simulink model "fourteen_bus_linear_network"  (R2020b)
settings: Solver=VariableStepAuto  StartTime=0.0  StopTime=1.000000  RelTol=1e-3
libraries: powerlib x124, powerlib_meascontrol x2
(part 2 of 2)

== system fourteen_bus_linear_network/Subsystem6 ==
  From Workspace15 : FromWorkspace  VariableName=load14_Ia_ts
  From Workspace16 : FromWorkspace  VariableName=load14_Ib_ts
  From Workspace17 : FromWorkspace  VariableName=load14_Ic_ts
  Subsystem3 : Subsystem
  A : PMIOPort  Side=Right
  B : PMIOPort  Port=2  Side=Right
  C : PMIOPort  Port=3  Side=Right
  wires:
  From Workspace15/1 -> Subsystem3/1(Ia)
  From Workspace17/1 -> Subsystem3/3(Ic)
  From Workspace16/1 -> Subsystem3/2(Ib)
  connections:
  Subsystem3/RConn2 -- B/RConn1
  Subsystem3/RConn1 -- A/RConn1
  Subsystem3/RConn3 -- C/RConn1

== system fourteen_bus_linear_network/Subsystem7 ==
  From Workspace15 : FromWorkspace  VariableName=load6_Ia_ts
  From Workspace16 : FromWorkspace  VariableName=load6_Ib_ts
  From Workspace17 : FromWorkspace  VariableName=load6_Ic_ts
  Subsystem3 : Subsystem
  A : PMIOPort  Side=Right
  B : PMIOPort  Port=2  Side=Right
  C : PMIOPort  Port=3  Side=Right
  wires:
  From Workspace15/1 -> Subsystem3/1(Ia)
  From Workspace17/1 -> Subsystem3/3(Ic)
  From Workspace16/1 -> Subsystem3/2(Ib)
  connections:
  Subsystem3/RConn2 -- B/RConn1
  Subsystem3/RConn1 -- A/RConn1
  Subsystem3/RConn3 -- C/RConn1

== system fourteen_bus_linear_network/Subsystem8 ==
  From Workspace15 : FromWorkspace  VariableName=load13_Ia_ts
  From Workspace16 : FromWorkspace  VariableName=load13_Ib_ts
  From Workspace17 : FromWorkspace  VariableName=load13_Ic_ts
  Subsystem3 : Subsystem
  A : PMIOPort  Side=Right
  B : PMIOPort  Port=2  Side=Right
  C : PMIOPort  Port=3  Side=Right
  wires:
  From Workspace15/1 -> Subsystem3/1(Ia)
  From Workspace17/1 -> Subsystem3/3(Ic)
  From Workspace16/1 -> Subsystem3/2(Ib)
  connections:
  Subsystem3/RConn2 -- B/RConn1
  Subsystem3/RConn1 -- A/RConn1
  Subsystem3/RConn3 -- C/RConn1

== system fourteen_bus_linear_network/Subsystem9 ==
  From Workspace15 : FromWorkspace  VariableName=load12_Ia_ts
  From Workspace16 : FromWorkspace  VariableName=load12_Ib_ts
  From Workspace17 : FromWorkspace  VariableName=load12_Ic_ts
  Subsystem3 : Subsystem
  A : PMIOPort  Side=Right
  B : PMIOPort  Port=2  Side=Right
  C : PMIOPort  Port=3  Side=Right
  wires:
  From Workspace15/1 -> Subsystem3/1(Ia)
  From Workspace17/1 -> Subsystem3/3(Ic)
  From Workspace16/1 -> Subsystem3/2(Ib)
  connections:
  Subsystem3/RConn2 -- B/RConn1
  Subsystem3/RConn1 -- A/RConn1
  Subsystem3/RConn3 -- C/RConn1

== system fourteen_bus_linear_network/Subsystem1/Subsystem1 ==
  Ia : Inport
  Ib : Inport  Port=2
  Ic : Inport  Port=3
  Controlled Current Source10 : powerlib/Electrical Sources/Controlled Current Source  Initialize=on  Source_Type=AC  Amplitude=0  Phase=0  Frequency=0  Measurements=None
  Controlled Current Source11 : powerlib/Electrical Sources/Controlled Current Source  Initialize=on  Source_Type=AC  Amplitude=0  Phase=0  Frequency=0  Measurements=None
  Controlled Current Source9 : powerlib/Electrical Sources/Controlled Current Source  Initialize=on  Source_Type=AC  Amplitude=0  Phase=0  Frequency=0  Measurements=None
  Ground2 : powerlib/Elements/Ground  LConnTagsString=a
  A : PMIOPort  Side=Right
  B : PMIOPort  Port=2  Side=Right
  C : PMIOPort  Port=3  Side=Right
  wires:
  Ia/1 -> Controlled Current Source9/1
  Ic/1 -> Controlled Current Source11/1
  Ib/1 -> Controlled Current Source10/1
  connections:
  Controlled Current Source10/RConn1 -- B/RConn1
  Controlled Current Source9/RConn1 -- A/RConn1
  Controlled Current Source11/RConn1 -- C/RConn1
  Controlled Current Source11/LConn1 -- Controlled Current Source10/LConn1 -- Controlled Current Source9/LConn1 -- Ground2/LConn1

== system fourteen_bus_linear_network/Subsystem10/Subsystem3 ==
  Ia : Inport
  Ib : Inport  Port=2
  Ic : Inport  Port=3
  Controlled Current Source10 : powerlib/Electrical Sources/Controlled Current Source  Initialize=on  Source_Type=AC  Amplitude=0  Phase=0  Frequency=0  Measurements=None
  Controlled Current Source11 : powerlib/Electrical Sources/Controlled Current Source  Initialize=on  Source_Type=AC  Amplitude=0  Phase=0  Frequency=0  Measurements=None
  Controlled Current Source9 : powerlib/Electrical Sources/Controlled Current Source  Initialize=on  Source_Type=AC  Amplitude=0  Phase=0  Frequency=0  Measurements=None
  Ground2 : powerlib/Elements/Ground  LConnTagsString=a
  A : PMIOPort  Side=Right
  B : PMIOPort  Port=2  Side=Right
  C : PMIOPort  Port=3  Side=Right
  wires:
  Ia/1 -> Controlled Current Source9/1
  Ic/1 -> Controlled Current Source11/1
  Ib/1 -> Controlled Current Source10/1
  connections:
  Controlled Current Source10/RConn1 -- B/RConn1
  Controlled Current Source9/RConn1 -- A/RConn1
  Controlled Current Source11/RConn1 -- C/RConn1
  Controlled Current Source10/LConn1 -- Controlled Current Source11/LConn1 -- Controlled Current Source9/LConn1 -- Ground2/LConn1

== system fourteen_bus_linear_network/Subsystem11/Subsystem3 ==
  Ia : Inport
  Ib : Inport  Port=2
  Ic : Inport  Port=3
  Controlled Current Source10 : powerlib/Electrical Sources/Controlled Current Source  Initialize=on  Source_Type=AC  Amplitude=0  Phase=0  Frequency=0  Measurements=None
  Controlled Current Source11 : powerlib/Electrical Sources/Controlled Current Source  Initialize=on  Source_Type=AC  Amplitude=0  Phase=0  Frequency=0  Measurements=None
  Controlled Current Source9 : powerlib/Electrical Sources/Controlled Current Source  Initialize=on  Source_Type=AC  Amplitude=0  Phase=0  Frequency=0  Measurements=None
  Ground2 : powerlib/Elements/Ground  LConnTagsString=a
  A : PMIOPort  Side=Right
  B : PMIOPort  Port=2  Side=Right
  C : PMIOPort  Port=3  Side=Right
  wires:
  Ia/1 -> Controlled Current Source9/1
  Ic/1 -> Controlled Current Source11/1
  Ib/1 -> Controlled Current Source10/1
  connections:
  Controlled Current Source10/RConn1 -- B/RConn1
  Controlled Current Source9/RConn1 -- A/RConn1
  Controlled Current Source11/RConn1 -- C/RConn1
  Controlled Current Source10/LConn1 -- Controlled Current Source11/LConn1 -- Controlled Current Source9/LConn1 -- Ground2/LConn1

== system fourteen_bus_linear_network/Subsystem12/Subsystem1 ==
  Ia : Inport
  Ib : Inport  Port=2
  Ic : Inport  Port=3
  Controlled Current Source10 : powerlib/Electrical Sources/Controlled Current Source  Initialize=on  Source_Type=AC  Amplitude=0  Phase=0  Frequency=0  Measurements=None
  Controlled Current Source11 : powerlib/Electrical Sources/Controlled Current Source  Initialize=on  Source_Type=AC  Amplitude=0  Phase=0  Frequency=0  Measurements=None
  Controlled Current Source9 : powerlib/Electrical Sources/Controlled Current Source  Initialize=on  Source_Type=AC  Amplitude=0  Phase=0  Frequency=0  Measurements=None
  Ground2 : powerlib/Elements/Ground  LConnTagsString=a
  A : PMIOPort  Side=Right
  B : PMIOPort  Port=2  Side=Right
  C : PMIOPort  Port=3  Side=Right
  wires:
  Ia/1 -> Controlled Current Source9/1
  Ic/1 -> Controlled Current Source11/1
  Ib/1 -> Controlled Current Source10/1
  connections:
  Controlled Current Source10/RConn1 -- B/RConn1
  Controlled Current Source9/RConn1 -- A/RConn1
  Controlled Current Source11/RConn1 -- C/RConn1
  Controlled Current Source11/LConn1 -- Ground2/LConn1 -- Controlled Current Source10/LConn1 -- Controlled Current Source9/LConn1

== system fourteen_bus_linear_network/Subsystem13/Subsystem1 ==
  Ia : Inport
  Ib : Inport  Port=2
  Ic : Inport  Port=3
  Controlled Current Source10 : powerlib/Electrical Sources/Controlled Current Source  Initialize=on  Source_Type=AC  Amplitude=0  Phase=0  Frequency=0  Measurements=None
  Controlled Current Source11 : powerlib/Electrical Sources/Controlled Current Source  Initialize=on  Source_Type=AC  Amplitude=0  Phase=0  Frequency=0  Measurements=None
  Controlled Current Source9 : powerlib/Electrical Sources/Controlled Current Source  Initialize=on  Source_Type=AC  Amplitude=0  Phase=0  Frequency=0  Measurements=None
  Ground2 : powerlib/Elements/Ground  LConnTagsString=a
  A : PMIOPort  Side=Right
  B : PMIOPort  Port=2  Side=Right
  C : PMIOPort  Port=3  Side=Right
  wires:
  Ia/1 -> Controlled Current Source9/1
  Ic/1 -> Controlled Current Source11/1
  Ib/1 -> Controlled Current Source10/1
  connections:
  Controlled Current Source10/RConn1 -- B/RConn1
  Controlled Current Source9/RConn1 -- A/RConn1
  Controlled Current Source11/RConn1 -- C/RConn1
  Controlled Current Source11/LConn1 -- Controlled Current Source10/LConn1 -- Controlled Current Source9/LConn1 -- Ground2/LConn1

== system fourteen_bus_linear_network/Subsystem3/Subsystem3 ==
  Ia : Inport
  Ib : Inport  Port=2
  Ic : Inport  Port=3
  Controlled Current Source10 : powerlib/Electrical Sources/Controlled Current Source  Initialize=on  Source_Type=AC  Amplitude=0  Phase=0  Frequency=0  Measurements=None
  Controlled Current Source11 : powerlib/Electrical Sources/Controlled Current Source  Initialize=on  Source_Type=AC  Amplitude=0  Phase=0  Frequency=0  Measurements=None
  Controlled Current Source9 : powerlib/Electrical Sources/Controlled Current Source  Initialize=on  Source_Type=AC  Amplitude=0  Phase=0  Frequency=0  Measurements=None
  Ground2 : powerlib/Elements/Ground  LConnTagsString=a
  A : PMIOPort  Side=Right
  B : PMIOPort  Port=2  Side=Right
  C : PMIOPort  Port=3  Side=Right
  wires:
  Ia/1 -> Controlled Current Source9/1
  Ic/1 -> Controlled Current Source11/1
  Ib/1 -> Controlled Current Source10/1
  connections:
  Controlled Current Source10/RConn1 -- B/RConn1
  Controlled Current Source9/RConn1 -- A/RConn1
  Controlled Current Source11/RConn1 -- C/RConn1
  Controlled Current Source10/LConn1 -- Controlled Current Source11/LConn1 -- Controlled Current Source9/LConn1 -- Ground2/LConn1

== system fourteen_bus_linear_network/Subsystem4/Subsystem3 ==
  Ia : Inport
  Ib : Inport  Port=2
  Ic : Inport  Port=3
  Controlled Current Source10 : powerlib/Electrical Sources/Controlled Current Source  Initialize=on  Source_Type=AC  Amplitude=0  Phase=0  Frequency=0  Measurements=None
  Controlled Current Source11 : powerlib/Electrical Sources/Controlled Current Source  Initialize=on  Source_Type=AC  Amplitude=0  Phase=0  Frequency=0  Measurements=None
  Controlled Current Source9 : powerlib/Electrical Sources/Controlled Current Source  Initialize=on  Source_Type=AC  Amplitude=0  Phase=0  Frequency=0  Measurements=None
  Ground2 : powerlib/Elements/Ground  LConnTagsString=a
  A : PMIOPort  Side=Right
  B : PMIOPort  Port=2  Side=Right
  C : PMIOPort  Port=3  Side=Right
  wires:
  Ia/1 -> Controlled Current Source9/1
  Ic/1 -> Controlled Current Source11/1
  Ib/1 -> Controlled Current Source10/1
  connections:
  Controlled Current Source10/RConn1 -- B/RConn1
  Controlled Current Source9/RConn1 -- A/RConn1
  Controlled Current Source11/RConn1 -- C/RConn1
  Controlled Current Source10/LConn1 -- Controlled Current Source11/LConn1 -- Controlled Current Source9/LConn1 -- Ground2/LConn1

== system fourteen_bus_linear_network/Subsystem5/Subsystem3 ==
  Ia : Inport
  Ib : Inport  Port=2
  Ic : Inport  Port=3
  Controlled Current Source10 : powerlib/Electrical Sources/Controlled Current Source  Initialize=on  Source_Type=AC  Amplitude=0  Phase=0  Frequency=0  Measurements=None
  Controlled Current Source11 : powerlib/Electrical Sources/Controlled Current Source  Initialize=on  Source_Type=AC  Amplitude=0  Phase=0  Frequency=0  Measurements=None
  Controlled Current Source9 : powerlib/Electrical Sources/Controlled Current Source  Initialize=on  Source_Type=AC  Amplitude=0  Phase=0  Frequency=0  Measurements=None
  Ground2 : powerlib/Elements/Ground  LConnTagsString=a
  A : PMIOPort  Side=Right
  B : PMIOPort  Port=2  Side=Right
  C : PMIOPort  Port=3  Side=Right
  wires:
  Ia/1 -> Controlled Current Source9/1
  Ic/1 -> Controlled Current Source11/1
  Ib/1 -> Controlled Current Source10/1
  connections:
  Controlled Current Source10/RConn1 -- B/RConn1
  Controlled Current Source9/RConn1 -- A/RConn1
  Controlled Current Source11/RConn1 -- C/RConn1
  Controlled Current Source11/LConn1 -- Controlled Current Source10/LConn1 -- Ground2/LConn1 -- Controlled Current Source9/LConn1

== system fourteen_bus_linear_network/Subsystem6/Subsystem3 ==
  Ia : Inport
  Ib : Inport  Port=2
  Ic : Inport  Port=3
  Controlled Current Source10 : powerlib/Electrical Sources/Controlled Current Source  Initialize=on  Source_Type=AC  Amplitude=0  Phase=0  Frequency=0  Measurements=None
  Controlled Current Source11 : powerlib/Electrical Sources/Controlled Current Source  Initialize=on  Source_Type=AC  Amplitude=0  Phase=0  Frequency=0  Measurements=None
  Controlled Current Source9 : powerlib/Electrical Sources/Controlled Current Source  Initialize=on  Source_Type=AC  Amplitude=0  Phase=0  Frequency=0  Measurements=None
  Ground2 : powerlib/Elements/Ground  LConnTagsString=a
  A : PMIOPort  Side=Right
  B : PMIOPort  Port=2  Side=Right
  C : PMIOPort  Port=3  Side=Right
  wires:
  Ia/1 -> Controlled Current Source9/1
  Ic/1 -> Controlled Current Source11/1
  Ib/1 -> Controlled Current Source10/1
  connections:
  Controlled Current Source10/RConn1 -- B/RConn1
  Controlled Current Source9/RConn1 -- A/RConn1
  Controlled Current Source11/RConn1 -- C/RConn1
  Controlled Current Source10/LConn1 -- Controlled Current Source11/LConn1 -- Controlled Current Source9/LConn1 -- Ground2/LConn1

== system fourteen_bus_linear_network/Subsystem7/Subsystem3 ==
  Ia : Inport
  Ib : Inport  Port=2
  Ic : Inport  Port=3
  Controlled Current Source10 : powerlib/Electrical Sources/Controlled Current Source  Initialize=on  Source_Type=AC  Amplitude=0  Phase=0  Frequency=0  Measurements=None
  Controlled Current Source11 : powerlib/Electrical Sources/Controlled Current Source  Initialize=on  Source_Type=AC  Amplitude=0  Phase=0  Frequency=0  Measurements=None
  Controlled Current Source9 : powerlib/Electrical Sources/Controlled Current Source  Initialize=on  Source_Type=AC  Amplitude=0  Phase=0  Frequency=0  Measurements=None
  Ground2 : powerlib/Elements/Ground  LConnTagsString=a
  A : PMIOPort  Side=Right
  B : PMIOPort  Port=2  Side=Right
  C : PMIOPort  Port=3  Side=Right
  wires:
  Ia/1 -> Controlled Current Source9/1
  Ic/1 -> Controlled Current Source11/1
  Ib/1 -> Controlled Current Source10/1
  connections:
  Controlled Current Source10/RConn1 -- B/RConn1
  Controlled Current Source9/RConn1 -- A/RConn1
  Controlled Current Source11/RConn1 -- C/RConn1
  Controlled Current Source10/LConn1 -- Controlled Current Source11/LConn1 -- Controlled Current Source9/LConn1 -- Ground2/LConn1

== system fourteen_bus_linear_network/Subsystem8/Subsystem3 ==
  Ia : Inport
  Ib : Inport  Port=2
  Ic : Inport  Port=3
  Controlled Current Source10 : powerlib/Electrical Sources/Controlled Current Source  Initialize=on  Source_Type=AC  Amplitude=0  Phase=0  Frequency=0  Measurements=None
  Controlled Current Source11 : powerlib/Electrical Sources/Controlled Current Source  Initialize=on  Source_Type=AC  Amplitude=0  Phase=0  Frequency=0  Measurements=None
  Controlled Current Source9 : powerlib/Electrical Sources/Controlled Current Source  Initialize=on  Source_Type=AC  Amplitude=0  Phase=0  Frequency=0  Measurements=None
  Ground2 : powerlib/Elements/Ground  LConnTagsString=a
  A : PMIOPort  Side=Right
  B : PMIOPort  Port=2  Side=Right
  C : PMIOPort  Port=3  Side=Right
  wires:
  Ia/1 -> Controlled Current Source9/1
  Ic/1 -> Controlled Current Source11/1
  Ib/1 -> Controlled Current Source10/1
  connections:
  Controlled Current Source10/RConn1 -- B/RConn1
  Controlled Current Source9/RConn1 -- A/RConn1
  Controlled Current Source11/RConn1 -- C/RConn1
  Controlled Current Source10/LConn1 -- Controlled Current Source11/LConn1 -- Controlled Current Source9/LConn1 -- Ground2/LConn1

== system fourteen_bus_linear_network/Subsystem9/Subsystem3 ==
  Ia : Inport
  Ib : Inport  Port=2
  Ic : Inport  Port=3
  Controlled Current Source10 : powerlib/Electrical Sources/Controlled Current Source  Initialize=on  Source_Type=AC  Amplitude=0  Phase=0  Frequency=0  Measurements=None
  Controlled Current Source11 : powerlib/Electrical Sources/Controlled Current Source  Initialize=on  Source_Type=AC  Amplitude=0  Phase=0  Frequency=0  Measurements=None
  Controlled Current Source9 : powerlib/Electrical Sources/Controlled Current Source  Initialize=on  Source_Type=AC  Amplitude=0  Phase=0  Frequency=0  Measurements=None
  Ground2 : powerlib/Elements/Ground  LConnTagsString=a
  A : PMIOPort  Side=Right
  B : PMIOPort  Port=2  Side=Right
  C : PMIOPort  Port=3  Side=Right
  wires:
  Ia/1 -> Controlled Current Source9/1
  Ic/1 -> Controlled Current Source11/1
  Ib/1 -> Controlled Current Source10/1
  connections:
  Controlled Current Source10/RConn1 -- B/RConn1
  Controlled Current Source9/RConn1 -- A/RConn1
  Controlled Current Source11/RConn1 -- C/RConn1
  Controlled Current Source10/LConn1 -- Controlled Current Source11/LConn1 -- Controlled Current Source9/LConn1 -- Ground2/LConn1
